simulink model "Old_Determining_Forces_Mass"  (R2016a)
settings: Solver=VariableStepAuto  StartTime=0.0  StopTime=10.0  RelTol=1e-3
undefined symbols (not defined in the file or in its folder): g0, mass_0, mass_e, mass_f
settings Model: Creator=Bakry  LastModifiedBy=Bakry

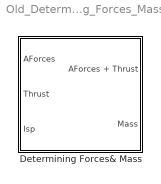
== system Old_Determining_Forces_Mass ==
  Determining Forces& Mass : Subsystem

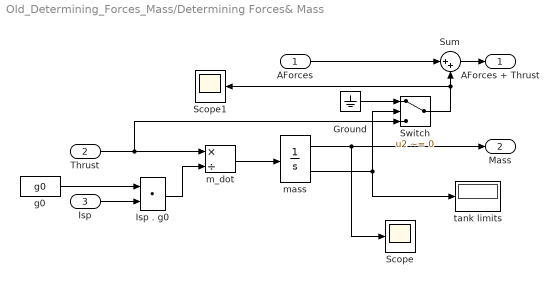
== system Old_Determining_Forces_Mass/Determining Forces& Mass ==
  AForces : Inport
  Thrust : Inport  Port=2
  Isp : Inport  Port=3
  Ground : Ground
  Isp . g0 : DotProduct  InputSameDT=on  OutDataTypeStr=Inherit: Inherit via internal rule
  Scope : Scope
  Scope1 : Scope
  Sum : Sum  Inputs=|++  SaturateOnIntegerOverflow=on
  Switch : Switch  Criteria=u2 ~= 0
  g0 : Constant  Value=g0
  m_dot : Product  Inputs=*/
  "mass  " : Integrator  InitialCondition=mass_0  LimitOutput=on  UpperSaturationLimit=mass_f  LowerSaturationLimit=mass_e  ShowSaturationPort=on
  tank limits : Display
  "AForces + Thrust " : Outport  PortDimensions=3
  Mass : Outport  Port=2
  wires:
  Thrust/1 -> Switch/3, m_dot/1
  Ground/1 -> Switch/1
  Switch/1 -> Scope1/1, Sum/2
  Sum/1 -> "AForces + Thrust "/1
  AForces/1 -> Sum/1
  m_dot/1 -> "mass  "/1
  "mass  "/2 -> tank limits/1, Switch/2
  Isp . g0/1 -> m_dot/2
  Isp/1 -> Isp . g0/2
  g0/1 -> Isp . g0/1
  "mass  "/1 -> Scope/1, Mass/1
